simulink model "method2"  (R2019b)
settings: Solver=VariableStepAuto  StartTime=0.0  StopTime=2  RelTol=1e-3
libraries: powerlib x23, simulink x2, powerlib_meascontrol x1
settings Model: Creator=96547  LastModifiedBy=96547
settings SolverCC: ZeroCrossAlgorithm=Adaptive
settings DataIOCC: ReturnWorkspaceOutputs=off
settings DebuggingCC: IgnoredZcDiagnostic=none

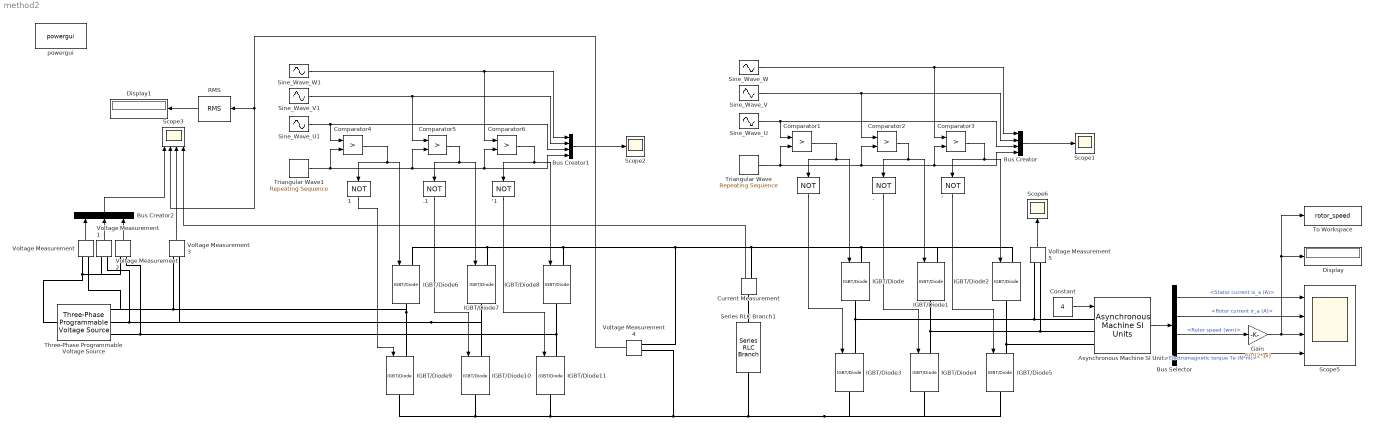
== system method2 ==
  " " : Logic  Operator=NOT  AllPortsSameDT=off  OutDataTypeStr=boolean
  " '" : Logic  Operator=NOT  AllPortsSameDT=off  OutDataTypeStr=boolean
  " '1" : Logic  Operator=NOT  AllPortsSameDT=off  OutDataTypeStr=boolean
  " ." : Logic  Operator=NOT  AllPortsSameDT=off  OutDataTypeStr=boolean
  " .1" : Logic  Operator=NOT  AllPortsSameDT=off  OutDataTypeStr=boolean
  " 1" : Logic  Operator=NOT  AllPortsSameDT=off  OutDataTypeStr=boolean
  Asynchronous Machine SI Units : powerlib/Machines/Asynchronous Machine SI Units  RotorType=Squirrel-cage  PresetModel=No  MechanicalLoad=Torque Tm  ShowDetailedParameters=on  ReferenceFrame=Stationary  Units=SI  MeasurementBus=off  NominalParameters=[ 3*800, 110, 50 ]  Stator="[ 0.635  1*2.0e-3 ]"  Rotor="[ 0.816  1.5e-3 ]"  Cage1=[0.4155 0.002066]  Cage2=[0.4168 0.0003495]  Lm=76.31e-3  Mechanical="[ 0.25  0 2]"  PolePairs=2  InitialConditions="[ 1,0   0,0,0   0,0,0 ]"  SimulateSaturation=off  Saturation=[14.03593122, 27.81365428, 53.79336849, 72.68890987, 97.98006896, 148.6815601, 215.7428561, 302.9841135, 428.7778367 ; 230, 322, 414, 460, 506, 552, 598, 644, 690]  LoadFlowParameters=1492000  TsPowergui=0  TsBlock=-1  IterativeModel=Trapezoidal non iterative  IterativeDiscreteModel=Trapezoidal non iterative  Pmec=0
      settings: SourceProductName=Simscape Electrical
  Bus Creator : BusCreator  DialogController=Simulink.DDGSource_Bus  Inputs=4
  Bus Creator1 : BusCreator  DialogController=Simulink.DDGSource_Bus  Inputs=4
  Bus Creator2 : BusCreator  DialogController=Simulink.DDGSource_Bus  Inputs=3
  Bus Selector : BusSelector  OutputSignals=Stator measurements.Stator current is_a (A),Rotor measurements.Rotor current ir_a (A),Mechanical.Rotor speed (wm),Mechanical.Electromagnetic torque Te (N*m)
  Comparator{1..6} (6 alike) : RelationalOperator  Operator=>  OutDataTypeStr=boolean  RndMeth=Nearest
  Constant : Constant  Value=4
  Current Measurement : powerlib/Measurements/Current Measurement  PhasorSimulation=off  OutputType=Complex  PSBequivalent=0
      settings: SourceProductName=Simscape Electrical
  Display : Display
  Display1 : Display
  Gain : Gain  Gain=60/(2*pi)
  IGBT/Diode{,1..11} (12 alike) : powerlib/Power Electronics/IGBT//Diode  Ron=1e-3  Rs=1e5  Cs=inf  Measurements=off
      settings: SourceProductName=Simscape Electrical
  RMS : powerlib_meascontrol/Measurements/RMS  TrueRMS=on  Freq=60  RMSInit=120  Ts=0
      settings: SourceProductName=Simscape Electrical
  Scope1 : Scope
  Scope2 : Scope
  Scope3 : Scope  NumInputPorts=4
  Scope5 : Scope  NumInputPorts=4
  Scope6 : Scope
  Series RLC Branch1 : powerlib/Elements/Series RLC Branch  LConnTagsString=__new0  RConnTagsString=__new0  BranchType=RC  Resistance=1e-6  Inductance=1e-3  SetiL0=off  InitialCurrent=0  Capacitance=1e-6  Setx0=off  InitialVoltage=0  Measurements=None
      settings: SourceProductName=Simscape Electrical
  Sine_Wave_U : Sin  Amplitude=0.8  Frequency=251  SampleTime=0
  Sine_Wave_U1 : Sin  Amplitude=0.8  Frequency=251  SampleTime=0
  Sine_Wave_V : Sin  Amplitude=0.8  Frequency=251  Phase=-2*pi/3  SampleTime=0
  Sine_Wave_V1 : Sin  Amplitude=0.8  Frequency=251  Phase=-2*pi/3  SampleTime=0
  Sine_Wave_W : Sin  Amplitude=0.8  Frequency=251  Phase=2*pi/3  SampleTime=0
  Sine_Wave_W1 : Sin  Amplitude=0.8  Frequency=251  Phase=2*pi/3  SampleTime=0
  Three-Phase Programmable Voltage Source : powerlib/Electrical Sources/Three-Phase Programmable Voltage Source  PositiveSequence="[110  0  40]"  VariationEntity=None  VariationType=Table of time-amplitude pairs  VariationTypeAlt=Step  VariationStep=0.5  VariationRate=10  VariationMagnitude=0.3  VariationFrequency=2  VariationTiming=[1 2]  VariationPhaseA=off  Amplitudes=[1 0.8 1.2 1.0]  TimeValues=[0 0.1 0.15 0.2]  HarmonicGeneration=off  HarmonicA=[3 0.2 -25 0]  HarmonicB=[2 0.15 35 2]  Timing="[0.05  3]"  BusType=swing  Pref=0  Qref=0  Qmin=-inf  Qmax=inf
      settings: SourceProductName=Simscape Electrical
  To Workspace : ToWorkspace  VariableName=rotor_speed  SampleTime=-1
      settings: Save2DSignal=2-D array (concatenate along first dimension)
  Triangular Wave : simulink/Sources/Repeating Sequence  rep_seq_t=[0 0.416e-5 0.833e-4 1.249e-4 1.667e-4]  rep_seq_y=[0 1 0 -1 0]
  Triangular Wave1 : simulink/Sources/Repeating Sequence  rep_seq_t=[0 0.416e-5 0.833e-4 1.249e-4 1.667e-4]  rep_seq_y=[0 1 0 -1 0]
  Voltage Measurement{,1..5} (6 alike) : powerlib/Measurements/Voltage Measurement  PhasorSimulation=off  OutputType=Complex  PSBequivalent=0
      settings: SourceProductName=Simscape Electrical
  powergui : powerlib/powergui  Priority=1  SimulationMode=Continuous  SampleTime=50e-6  frequency=60  Iterations=50  frequencyindice=50  Pbase=100e6  ErrMax=1e-4  UnitsV=kV  UnitsW=MW  buscounter=0  FunctionMessages=off  echomessages=off  EnableUseOfTLC=off  CurrentSourceSwitches=off  DisableSnubberDevices=off  DisableRonSwitches=off  DisableVfSwitches=off  DisplayEquations=off  AutomaticDiscreteSolvers=off  SolverType=Tustin/Backward Euler (TBE)  Interpol=off  ExternalGateDelay=off  methode=off  Ts=100  x0status=blocks  SPID=on  SwTol=0  HookPort=off  NonlinearTolerance=1e-4  nMaxIteration=100  ContinueOnMaxIteration=off  RestoreLinks=warning  ResistiveCurrentMeasurement=off  Frange=[0:2:500]  Ylog=off  Xlog=on  ShowGrid=off  save=off  variable=ZData  structure=0  ZoomFFT=off  StartTime=0.0  cycles=1  DisplayStyle=1  fundamental=60  FreqAxis=off  MaxFrequency=1000  frequencyindicesteady=1  RmsSteady=1  display=off
      settings: SourceProductName=Simscape Electrical
  wires:
  Sine_Wave_V/1 -> Comparator2/1, Bus Creator/2
  " '"/1 -> IGBT/Diode5/1
  Comparator3/1 -> IGBT/Diode2/1, " '"/1
  Sine_Wave_U/1 -> Bus Creator/3, Comparator1/1
  " ."/1 -> IGBT/Diode4/1
  " "/1 -> IGBT/Diode3/1
  Comparator2/1 -> IGBT/Diode1/1, " ."/1
  Triangular Wave/1 -> Comparator1/2, Comparator2/2, Comparator3/2, Bus Creator/4
  Sine_Wave_W/1 -> Comparator3/1, Bus Creator/1
  Comparator1/1 -> " "/1, IGBT/Diode/1
  Bus Creator/1 -> Scope1/1
  Voltage Measurement/1 -> Bus Creator2/1
  Voltage Measurement1/1 -> Bus Creator2/2
  Voltage Measurement2/1 -> Bus Creator2/3
  Bus Creator2/1 -> Scope3/1
  Voltage Measurement3/1 -> Scope3/3
  Voltage Measurement4/1 -> Scope3/2, RMS/1
  Constant/1 -> Asynchronous Machine SI Units/1
  Voltage Measurement5/1 -> Scope6/1
  Bus Selector/1 -> Scope5/1  "<Stator current is_a (A)>"
  Bus Selector/2 -> Scope5/2  "<Rotor current ir_a (A)>"
  Bus Selector/4 -> Scope5/4  "<Electromagnetic torque Te (N*m)>"
  Asynchronous Machine SI Units/1 -> Bus Selector/1
  Bus Selector/3 -> Gain/1  "<Rotor speed (wm)>"
  Gain/1 -> To Workspace/1, Display/1, Scope5/3
  Current Measurement/1 -> Scope3/4
  RMS/1 -> Display1/1
  Comparator4/1 -> IGBT/Diode6/1, " 1"/1
  Sine_Wave_W1/1 -> Bus Creator1/1, Comparator6/1
  Triangular Wave1/1 -> Bus Creator1/4, Comparator6/2, Comparator5/2, Comparator4/2
  Comparator5/1 -> " .1"/1, IGBT/Diode7/1
  " 1"/1 -> IGBT/Diode9/1
  " .1"/1 -> IGBT/Diode10/1
  Sine_Wave_U1/1 -> Comparator4/1, Bus Creator1/3
  Comparator6/1 -> " '1"/1, IGBT/Diode8/1
  " '1"/1 -> IGBT/Diode11/1
  Sine_Wave_V1/1 -> Bus Creator1/2, Comparator5/1
  Bus Creator1/1 -> Scope2/1
  connections:
  IGBT/Diode3/LConn1 -- IGBT/Diode/RConn1 -- Asynchronous Machine SI Units/LConn1 -- Voltage Measurement5/LConn1
  IGBT/Diode8/LConn1 -- IGBT/Diode7/LConn1 -- IGBT/Diode6/LConn1 -- IGBT/Diode2/LConn1 -- IGBT/Diode1/LConn1 -- IGBT/Diode/LConn1 -- Current Measurement/RConn1 -- Voltage Measurement4/LConn2
  IGBT/Diode9/RConn1 -- IGBT/Diode10/RConn1 -- IGBT/Diode11/RConn1 -- IGBT/Diode3/RConn1 -- IGBT/Diode4/RConn1 -- IGBT/Diode5/RConn1 -- Series RLC Branch1/RConn1 -- Voltage Measurement4/LConn1
  IGBT/Diode4/LConn1 -- IGBT/Diode1/RConn1 -- Asynchronous Machine SI Units/LConn2 -- Voltage Measurement5/LConn2
  IGBT/Diode5/LConn1 -- Asynchronous Machine SI Units/LConn3 -- IGBT/Diode2/RConn1
  IGBT/Diode9/LConn1 -- IGBT/Diode6/RConn1 -- Voltage Measurement/LConn2 -- Three-Phase Programmable Voltage Source/RConn1 -- Voltage Measurement3/LConn1
  Voltage Measurement2/LConn2 -- Three-Phase Programmable Voltage Source/RConn3 -- IGBT/Diode11/LConn1 -- IGBT/Diode8/RConn1
  Voltage Measurement/LConn1 -- Three-Phase Programmable Voltage Source/LConn1 -- Voltage Measurement2/LConn1 -- Voltage Measurement1/LConn1
  Current Measurement/LConn1 -- Series RLC Branch1/LConn1
  Three-Phase Programmable Voltage Source/RConn2 -- IGBT/Diode10/LConn1 -- IGBT/Diode7/RConn1 -- Voltage Measurement3/LConn2 -- Voltage Measurement1/LConn2
